simulink model "simulate_passbandEnvelope_AM"  (R2017a)
settings: Solver=VariableStepAuto  StartTime=0.0  StopTime=.1  RelTol=1e-3
InitFcn:
  | fs = 1e4;
  | frameSize = 1000;
libraries: dspsrcs4 x3
settings Model: Creator=prust  LastModifiedBy=prust

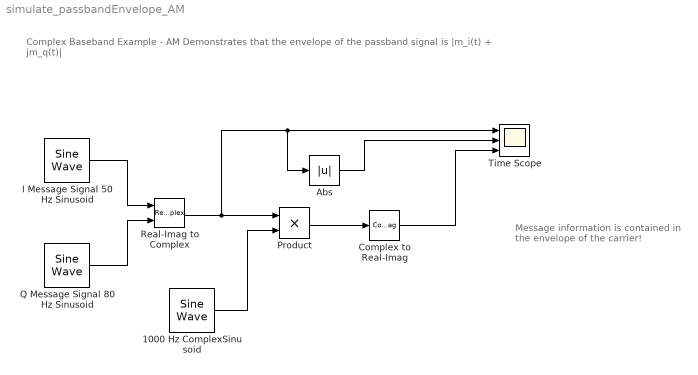
== system simulate_passbandEnvelope_AM ==
  note: Message information is contained
      | in the envelope of the carrier!
  note: Complex Baseband Example - AM
      | Demonstrates that the envelope of the passband signal is |m_i(t) + jm_q(t)|
  1000 Hz ComplexSinusoid : dspsrcs4/Sine Wave  Amplitude=sqrt(2)  Frequency=1000  Phase=0  SampleMode=Discrete  OutComplex=Complex  CompMethod=Trigonometric fcn  TableSize=Speed  SampleTime=1/fs  SamplesPerFrame=frameSize  ResetState=Restart at time zero  OutputFrames=off  dataType=double  wordLen=16  udDataType=sfix(16)  fracBitsMode=Best precision  numFracBits=15  OutDataTypeStr=double  LastOutDataTypeStr=double
  Abs : Abs
  Complex to Real-Imag : ComplexToRealImag  Output=Real
  I Message Signal 50 Hz Sinusoid : dspsrcs4/Sine Wave  Amplitude=1  Frequency=50  Phase=0  SampleMode=Discrete  OutComplex=Real  CompMethod=Trigonometric fcn  TableSize=Speed  SampleTime=1/fs  SamplesPerFrame=frameSize  ResetState=Restart at time zero  OutputFrames=off  dataType=double  wordLen=16  udDataType=sfix(16)  fracBitsMode=Best precision  numFracBits=15  OutDataTypeStr=double  LastOutDataTypeStr=double
  Product : Product
  Q Message Signal 80 Hz Sinusoid : dspsrcs4/Sine Wave  Amplitude=1  Frequency=80  Phase=0  SampleMode=Discrete  OutComplex=Real  CompMethod=Trigonometric fcn  TableSize=Speed  SampleTime=1/fs  SamplesPerFrame=frameSize  ResetState=Restart at time zero  OutputFrames=off  dataType=double  wordLen=16  udDataType=sfix(16)  fracBitsMode=Best precision  numFracBits=15  OutDataTypeStr=double  LastOutDataTypeStr=double
  Real-Imag to Complex : RealImagToComplex
  Time Scope : Scope  NumInputPorts=3
  wires:
  I Message Signal 50 Hz Sinusoid/1 -> Real-Imag to Complex/1
  Q Message Signal 80 Hz Sinusoid/1 -> Real-Imag to Complex/2
  Real-Imag to Complex/1 -> Abs/1, Time Scope/1, Product/1
  1000 Hz ComplexSinusoid/1 -> Product/2
  Product/1 -> Complex to Real-Imag/1
  Abs/1 -> Time Scope/2
  Complex to Real-Imag/1 -> Time Scope/3
